simulink model "inner_PD_c"  (Simulink 8.7)
settings: Solver=VariableStepAuto  StartTime=0.0  StopTime=10  RelTol=1e-3
undefined symbols (not defined in the file or in its folder): g, I, KetaD, KetaP, KzD, KzP, m
settings Model: Creator=Daniel  LastModifiedBy=mgreiff
settings DataIOCC: SaveFormat=Dataset
settings DebuggingCC: UnderspecifiedInitializationDetection=Simplified  MergeDetectMultiDrivingBlocksExec=error  AllowSymbolicDim=off
settings HardwareCC: ProdBitPerPointer=64  ProdLargestAtomicFloat=Float  ProdIntDivRoundTo=Zero  ProdEndianess=LittleEndian  ProdWordSize=64  ProdHWDeviceType=Intel->x86-64 (Windows64)
settings GRTTargetCC: GeneratePreprocessorConditionals=Use local settings
settings ConfigComp: CovModelRefEnable=off

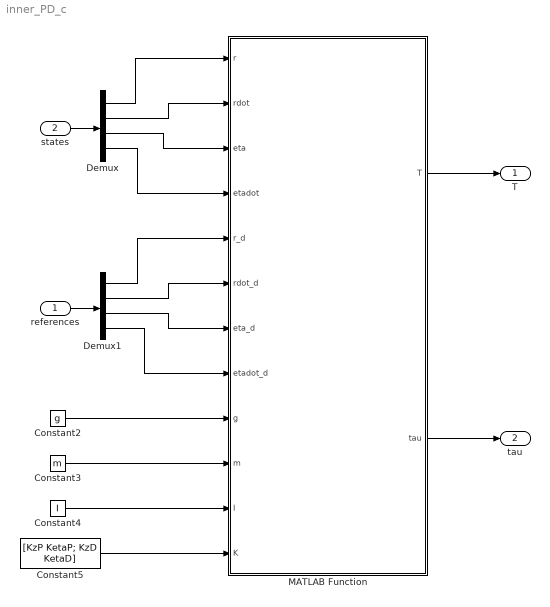
== system inner_PD_c ==
  references : Inport  PortDimensions=12
  states : Inport  Port=2  PortDimensions=12
  Constant2 : Constant  Value=g
  Constant3 : Constant  Value=m
  Constant4 : Constant  Value=I
  Constant5 : Constant  Value=[KzP KetaP; KzD KetaD]
  Demux : Demux  Outputs=[3,3,3,3]
  Demux1 : Demux  Outputs=[3,3,3,3]
  MATLAB Function : MATLAB Function  TreatAsAtomicUnit=on
      settings: MinAlgLoopOccurrences=on
  T : Outport  PortDimensions=1
  tau : Outport  Port=2  PortDimensions=3
  wires:
  Demux/2 -> MATLAB Function/2(rdot)
  Demux/4 -> MATLAB Function/4(etadot)
  Demux1/2 -> MATLAB Function/6(rdot_d)
  Demux1/4 -> MATLAB Function/8(etadot_d)
  Constant2/1 -> MATLAB Function/9(g)
  Constant4/1 -> MATLAB Function/11(I)
  Constant3/1 -> MATLAB Function/10(m)
  Constant5/1 -> MATLAB Function/12(K)
  MATLAB Function/1(T) -> T/1
  states/1 -> Demux/1
  Demux/1 -> MATLAB Function/1(r)
  Demux/3 -> MATLAB Function/3(eta)
  references/1 -> Demux1/1
  Demux1/1 -> MATLAB Function/5(r_d)
  Demux1/3 -> MATLAB Function/7(eta_d)
  MATLAB Function/2(tau) -> tau/1

== matlab function MATLAB Function ==
  data: r input double; rdot input double; T output double; eta input double; etadot input double; r_d input double; rdot_d input double; eta_d input double; etadot_d input double; g input double; m input double; I input double; K input double; tau output double
function [T, tau] = copter_PD(r, rdot, eta, etadot, r_d, rdot_d, eta_d, etadot_d, g, m, I, K)
    KzP = K(1,1); KetaP = K(1,2:4)';
    KzD = K(2,1); KetaD = K(2,2:4)';
    
    phi = eta(1); theta = eta(2);
    
    T = m/(cos(phi)*cos(theta)) * (g + KzD * (rdot_d(3) - rdot(3)) + KzP * (r_d(3) - r(3)));
    tau = diag(I) * (KetaD .* (etadot_d - etadot) + KetaP .* (eta_d - eta));
end
